simulink model "P_Respuesta_Ideal_Labierto"  (R2021b)
settings: Solver=VariableStepAuto  StartTime=0.0  StopTime=20  RelTol=1e-3
libraries: fl_lib x6, nesl_utility x3
settings Model: Creator=parra  LastModifiedBy=parra

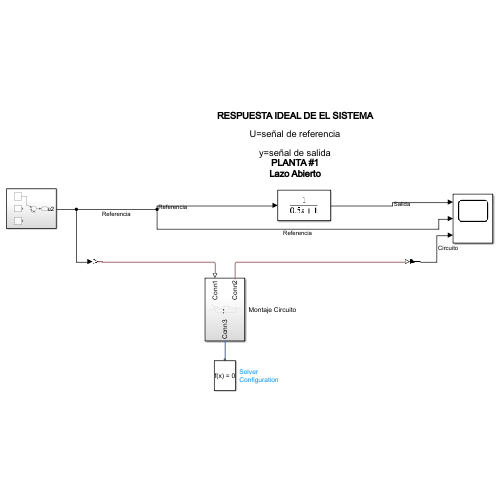
[thumbnail: Simulink's stored preview of the top-level diagram]
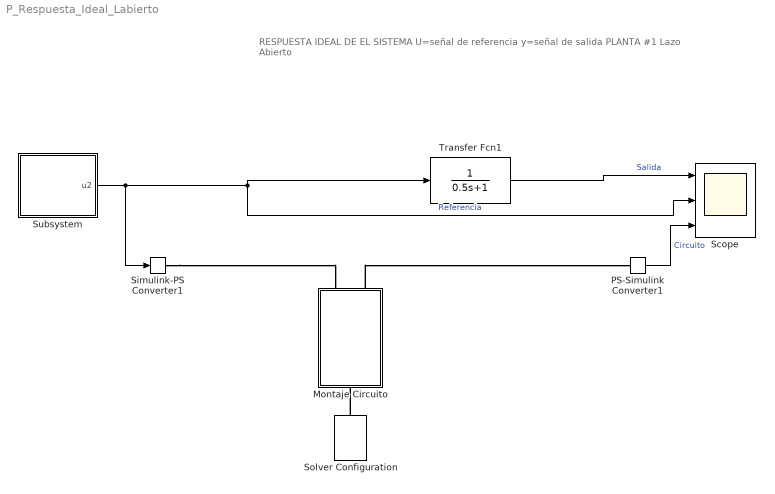
== system P_Respuesta_Ideal_Labierto ==
  note: RESPUESTA IDEAL DE EL SISTEMA
      |
      | U=señal de referencia
      |
      | y=señal de salida
      | PLANTA #1
      | Lazo Abierto
  Montaje Circuito : Subsystem
  PS-Simulink Converter1 : nesl_utility/PS-Simulink Converter  PhysicalDomain=network_engine_domain  SubClassName=ps_output  LeftPortType=input  RightPortType=output  PseudoPeriodic=off  Frequencies=[]  Unit=inherit  AffineConversion=off
      settings: SourceProductBaseCode=PW,SS
  Scope : Scope  NumInputPorts=3
  Simulink-PS Converter1 : nesl_utility/Simulink-PS Converter  PhysicalDomain=network_engine_domain  SubClassName=ps_input  LeftPortType=input  RightPortType=output  PseudoPeriodic=off  Frequencies=[]  NoiseDistribution=none  NoiseParameters=[]  Unit=1  AffineConversion=off  FilteringAndDerivatives=provide  SimscapeFilterOrder=1  InputFilterTimeConstant=0.001  UdotUserProvided=0
      settings: SourceProductBaseCode=PW,SS
  Solver Configuration : nesl_utility/Solver Configuration  PhysicalDomain=network_engine_domain  SubClassName=solver  LeftPortType=input  RightPortType=generic  Tones=[]  Harmonics=[]  SimulateNoise=off  Profile=off  UseLocalSampling=off  EnableSwitchedLinearOptims=on  FrequencyDomain=off  UseCCode=off  RelTol=0.001  AbsTol=0.001  MinStep=1e-09  ToWorkspace=off  RevertToSquareIcSolve=off  NumHomotopyIterations=100  PhasorMode=off  PhasorModeNumHarmonics=1  DoDC=off  ResidualTolerance=1e-09  UseLocalSolver=off  LocalSolverChoice=NE_BACKWARD_EULER_ADVANCER  LocalSolverSampleTime=0.001  DoFixedCost=off  MaxNonlinIter=3  MaxModeIter=2  ComputeImpulses=off  ImpulseIterations=2  LinearAlgebra=auto  EquationFormulation=NE_TIME_EF  DelaysMemoryBudget=1024  AutomaticFiltering=on  FilteringTimeConstant=0.001  PartitionStorageMethod=AS_NEEDED  PartitionMemoryBudget=1024  PartitionMethod=ROBUST
      settings: SourceProductBaseCode=PW,SS
  Subsystem : Subsystem
  Transfer Fcn1 : TransferFcn  Denominator=[0.5 1]
  wires:
  Subsystem/1(u2) -> Simulink-PS Converter1/1, Transfer Fcn1/1, Scope/2  "Referencia"
  Transfer Fcn1/1 -> Scope/1  "Salida"
  PS-Simulink Converter1/1 -> Scope/3  "Circuito"
  connections:
  Simulink-PS Converter1/RConn1 -- Montaje Circuito/RConn1
  Montaje Circuito/RConn2 -- PS-Simulink Converter1/LConn1
  Solver Configuration/RConn1 -- Montaje Circuito/LConn1

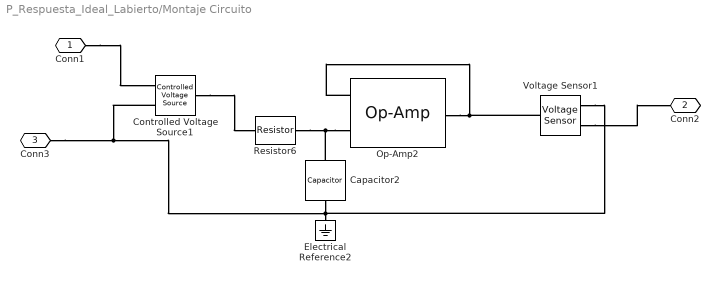
== system P_Respuesta_Ideal_Labierto/Montaje Circuito ==
  Capacitor2 : fl_lib/Electrical/Electrical Elements/Capacitor  c=10 uF  r=1e-6 Ohm  g=0 1/Ohm  i_specify=off  i_priority=None  i=0 A  i_nominal_specify=off  i_nominal_unit=A  i_nominal_value=1  v_specify=off  v_priority=None  v=0 V  v_nominal_specify=off  v_nominal_unit=V  v_nominal_value=1  vc_specify=off  vc_priority=High  vc=0 V  vc_nominal_specify=off  vc_nominal_unit=V  vc_nominal_value=1
  Controlled Voltage Source1 : fl_lib/Electrical/Electrical Sources/Controlled Voltage Source
  Electrical Reference2 : fl_lib/Electrical/Electrical Elements/Electrical Reference
  Op-Amp2 : fl_lib/Electrical/Electrical Elements/Op-Amp  outI_specify=off  outI_priority=None  outI=0 A  outI_nominal_specify=off  outI_nominal_unit=A  outI_nominal_value=1
  Resistor6 : fl_lib/Electrical/Electrical Elements/Resistor  R=50 kOhm  i_specify=off  i_priority=None  i=0 A  i_nominal_specify=off  i_nominal_unit=A  i_nominal_value=1  v_specify=off  v_priority=None  v=0 V  v_nominal_specify=off  v_nominal_unit=V  v_nominal_value=1
  Voltage Sensor1 : fl_lib/Electrical/Electrical Sensors/Voltage Sensor
  Conn1 : PMIOPort  Side=Right
  Conn2 : PMIOPort  Port=2  Side=Right
  Conn3 : PMIOPort  Port=3  Side=Left
  connections:
  Capacitor2/RConn1 -- Voltage Sensor1/RConn2 -- Conn3/RConn1 -- Controlled Voltage Source1/RConn2 -- Electrical Reference2/LConn1
  Conn1/RConn1 -- Controlled Voltage Source1/RConn1
  Voltage Sensor1/LConn1 -- Op-Amp2/LConn2 -- Op-Amp2/RConn1
  Op-Amp2/LConn1 -- Capacitor2/LConn1 -- Resistor6/RConn1
  Controlled Voltage Source1/LConn1 -- Resistor6/LConn1
  Voltage Sensor1/RConn1 -- Conn2/RConn1

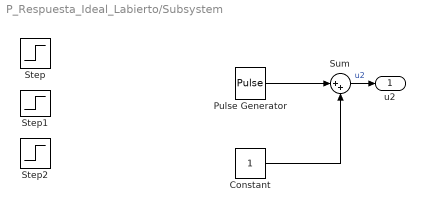
== system P_Respuesta_Ideal_Labierto/Subsystem ==
  Constant : Constant
  Pulse Generator : DiscretePulseGenerator  Amplitude=0.5  Period=2500  PulseWidth=1250  SampleTime=0.01
  Step : Step  Time=10  SampleTime=0.01
  Step1 : Step  Time=13  Before=1  After=1.5  SampleTime=0.01
  Step2 : Step  Time=16  Before=1  After=1.5  SampleTime=0.01
  Sum : Sum  Inputs=|++
  u2 : Outport
  wires:
  Sum/1 -> u2/1  "u2"
  Pulse Generator/1 -> Sum/1
  Constant/1 -> Sum/2
